simulink model "CIC"  (R2018a)
settings: Solver=ode45  StartTime=0.0  StopTime=Tsim  RelTol=1e-3  EnableMultiTasking=on
values from neighbouring files (symbols this model uses):
  Fin = 15    [Test_CIC.m]
  fo = 10    [Test_CIC.m]
  fsL = 50    [Test_CIC.m]
  M = 1    [Test_CIC.m]
  R = 2000    [Test_CIC.m]
  sel_b = [0 0]    [Test_CIC.m]
  Wg = 22    [Test_CIC.m]
libraries: dspsigops x3, dspsrcs4 x2
settings Model: Creator=jvalls  LastModifiedBy=gsandar
settings DataIOCC: LimitDataPoints=on  SaveFormat=Array  SignalLoggingSaveFormat=ModelDataLogs
settings OptimizationCC: ExpressionDepthLimit=2147483647  LifeSpan=inf
settings DebuggingCC: UnderspecifiedInitializationDetection=Classic  MergeDetectMultiDrivingBlocksExec=none  SolverPrmCheckMsg=warning  ParameterPrecisionLossMsg=none  FcnCallInpInsideContextMsg=warning  StateNameClashWarn=warning  SFUnexpectedBacktrackingDiag=warning  SFNoUnconditionalDefaultTransitionDiag=warning
settings HardwareCC: ProdBitPerPointer=32  ProdBitPerSizeT=32  ProdBitPerPtrDiffT=32  ProdLargestAtomicFloat=None  ProdIntDivRoundTo=Undefined  ProdEndianess=Unspecified  ProdWordSize=32  ProdHWDeviceType=32-bit Generic
settings ModelReferenceCC: PropagateSignalLabelsOutOfModel=off
settings CodeAppCC: StateflowObjectComments=on
settings GRTTargetCC: TargetLangStandard=C89/C90 (ANSI)  CombineOutputUpdateFcns=off  GRTInterface=on
settings ConfigComp: CovMetricSettings=dw  CovSaveCumulativeToWorkspaceVar=on  CovSaveSingleToWorkspaceVar=on  CovExternalEMLEnable=off  CovSFcnEnable=off

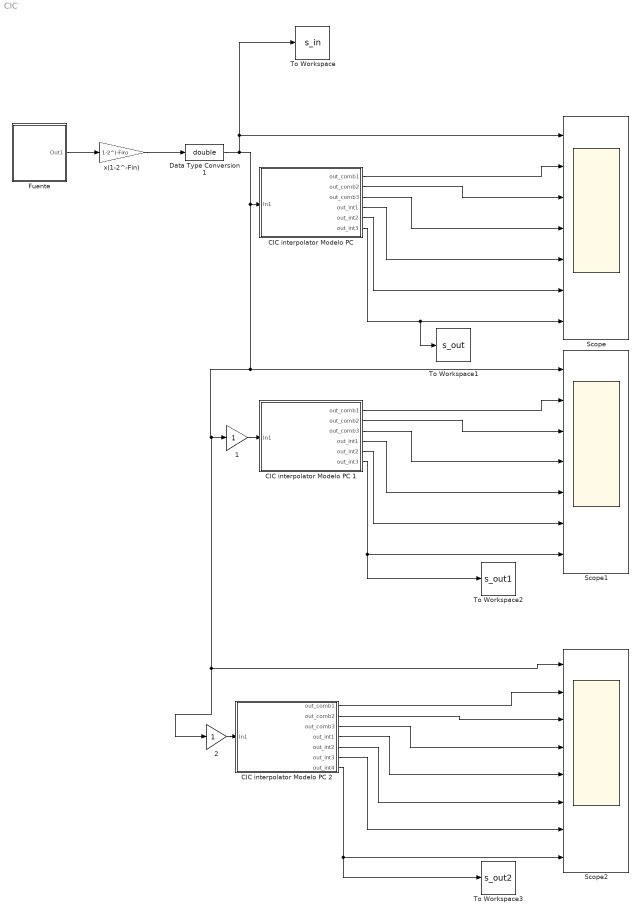
== system CIC ==
  1 : Gain  OutDataTypeStr=fixdt(1,Win,Fin)
  2 : Gain  OutDataTypeStr=fixdt(1,Win,Fin)
  "CIC interpolator Modelo PC " : Subsystem
  CIC interpolator Modelo PC 1 : Subsystem
  CIC interpolator Modelo PC 2 : Subsystem
  Data Type Conversion1 : DataTypeConversion  OutDataTypeStr=double
  Fuente : Subsystem
  Scope : Scope  NumInputPorts=7
  Scope1 : Scope  NumInputPorts=7
  Scope2 : Scope  NumInputPorts=8
  To Workspace : ToWorkspace  VariableName=s_in  SampleTime=-1
      settings: Save2DSignal=2-D array (concatenate along first dimension)
  To Workspace1 : ToWorkspace  VariableName=s_out  SampleTime=-1
      settings: Save2DSignal=2-D array (concatenate along first dimension)
  To Workspace2 : ToWorkspace  VariableName=s_out1  SampleTime=-1
      settings: Save2DSignal=2-D array (concatenate along first dimension)
  To Workspace3 : ToWorkspace  VariableName=s_out2  SampleTime=-1
      settings: Save2DSignal=2-D array (concatenate along first dimension)
  x(1-2^-Fin) : Gain  Gain=1-2^(-Fin)  OutDataTypeStr=fixdt(1,Win,Fin)
  wires:
  Data Type Conversion1/1 -> To Workspace/1, Scope/1, Scope2/1, 2/1, 1/1, Scope1/1, "CIC interpolator Modelo PC "/1(In1)
  Fuente/1(Out1) -> x(1-2^-Fin)/1
  x(1-2^-Fin)/1 -> Data Type Conversion1/1
  "CIC interpolator Modelo PC "/1(out_comb1) -> Scope/2
  "CIC interpolator Modelo PC "/2(out_comb2) -> Scope/3
  "CIC interpolator Modelo PC "/3(out_comb3) -> Scope/4
  "CIC interpolator Modelo PC "/4(out_int1) -> Scope/5
  "CIC interpolator Modelo PC "/5(out_int2) -> Scope/6
  "CIC interpolator Modelo PC "/6(out_int3) -> Scope/7, To Workspace1/1
  CIC interpolator Modelo PC 1/4(out_int1) -> Scope1/5
  CIC interpolator Modelo PC 1/2(out_comb2) -> Scope1/3
  CIC interpolator Modelo PC 1/6(out_int3) -> To Workspace2/1, Scope1/7
  CIC interpolator Modelo PC 1/3(out_comb3) -> Scope1/4
  CIC interpolator Modelo PC 1/1(out_comb1) -> Scope1/2
  CIC interpolator Modelo PC 1/5(out_int2) -> Scope1/6
  1/1 -> CIC interpolator Modelo PC 1/1(In1)
  2/1 -> CIC interpolator Modelo PC 2/1(In1)
  CIC interpolator Modelo PC 2/6(out_int3) -> Scope2/7
  CIC interpolator Modelo PC 2/5(out_int2) -> Scope2/6
  CIC interpolator Modelo PC 2/1(out_comb1) -> Scope2/2
  CIC interpolator Modelo PC 2/2(out_comb2) -> Scope2/3
  CIC interpolator Modelo PC 2/4(out_int1) -> Scope2/5
  CIC interpolator Modelo PC 2/3(out_comb3) -> Scope2/4
  CIC interpolator Modelo PC 2/7(out_int4) -> To Workspace3/1, Scope2/8

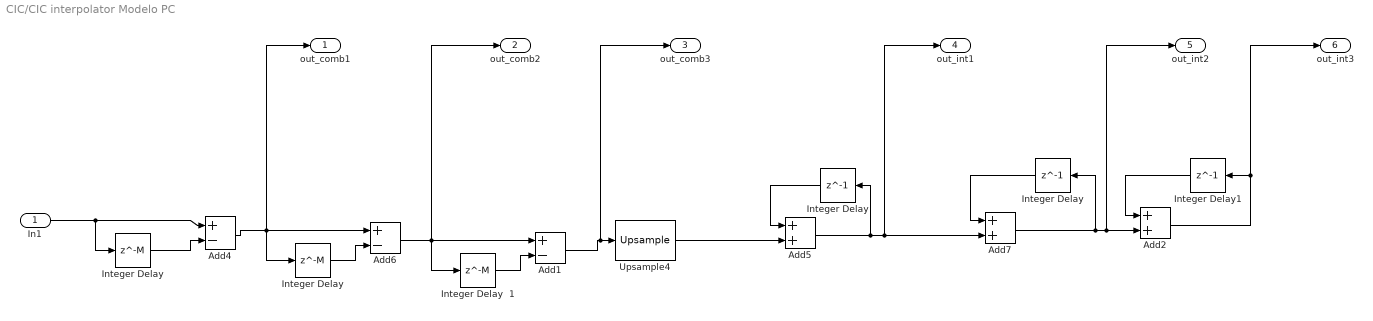
== system CIC/CIC interpolator Modelo PC  ==
  In1 : Inport
  " Integer Delay" : Delay  DelayLength=1
  " Integer Delay1" : Delay  DelayLength=1
  Add1 : Sum  Inputs=+-
  Add2 : Sum
  Add4 : Sum  Inputs=+-
  Add5 : Sum
  Add6 : Sum  Inputs=+-
  Add7 : Sum
  "Integer Delay " : Delay  DelayLength=1
  "Integer Delay " : Delay  DelayLength=M
  "Integer Delay  " : Delay  DelayLength=M
  Integer Delay  1 : Delay  DelayLength=M
  Upsample4 : dspsigops/Upsample  N=R  phase=0  InputProcessing=Columns as channels (frame based)  RateOptions=Allow multirate processing  ic=0  mode=Unused parameter value
  out_comb1 : Outport
  out_comb2 : Outport  Port=2
  out_comb3 : Outport  Port=3
  out_int1 : Outport  Port=4
  out_int2 : Outport  Port=5
  out_int3 : Outport  Port=6
  wires:
  In1/1 -> "Integer Delay "/1, Add4/1
  " Integer Delay"/1 -> Add7/1
  "Integer Delay "/1 -> Add5/1
  "Integer Delay "/1 -> Add4/2
  "Integer Delay  "/1 -> Add6/2
  Integer Delay  1/1 -> Add1/2
  " Integer Delay1"/1 -> Add2/1
  Upsample4/1 -> Add5/2
  Add6/1 -> out_comb2/1, Integer Delay  1/1, Add1/1
  Add4/1 -> out_comb1/1, "Integer Delay  "/1, Add6/1
  Add1/1 -> out_comb3/1, Upsample4/1
  Add5/1 -> "Integer Delay "/1, Add7/2, out_int1/1
  Add7/1 -> out_int2/1, Add2/2, " Integer Delay"/1
  Add2/1 -> out_int3/1, " Integer Delay1"/1

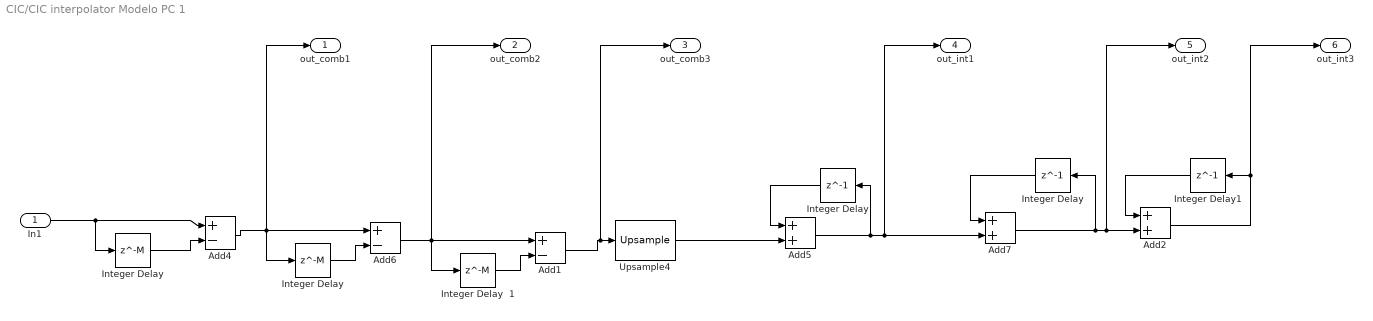
== system CIC/CIC interpolator Modelo PC 1 ==
  In1 : Inport
  " Integer Delay" : Delay  DelayLength=1
  " Integer Delay1" : Delay  DelayLength=1
  Add1 : Sum  Inputs=+-  OutDataTypeStr=fixdt(1,19,15)
  Add2 : Sum  OutDataTypeStr=fixdt(1,38,15)
  Add4 : Sum  Inputs=+-  OutDataTypeStr=fixdt(1,17,15)
  Add5 : Sum  OutDataTypeStr=fixdt(1,38,15)
  Add6 : Sum  Inputs=+-  OutDataTypeStr=fixdt(1,18,15)
  Add7 : Sum  OutDataTypeStr=fixdt(1,38,15)
  "Integer Delay " : Delay  DelayLength=1
  "Integer Delay " : Delay  DelayLength=M
  "Integer Delay  " : Delay  DelayLength=M
  Integer Delay  1 : Delay  DelayLength=M
  Upsample4 : dspsigops/Upsample  N=R  phase=0  InputProcessing=Columns as channels (frame based)  RateOptions=Allow multirate processing  ic=0  mode=Unused parameter value
  out_comb1 : Outport
  out_comb2 : Outport  Port=2
  out_comb3 : Outport  Port=3
  out_int1 : Outport  Port=4
  out_int2 : Outport  Port=5
  out_int3 : Outport  Port=6
  wires:
  In1/1 -> "Integer Delay "/1, Add4/1
  " Integer Delay"/1 -> Add7/1
  "Integer Delay "/1 -> Add5/1
  "Integer Delay "/1 -> Add4/2
  "Integer Delay  "/1 -> Add6/2
  Integer Delay  1/1 -> Add1/2
  " Integer Delay1"/1 -> Add2/1
  Upsample4/1 -> Add5/2
  Add6/1 -> out_comb2/1, Integer Delay  1/1, Add1/1
  Add4/1 -> out_comb1/1, "Integer Delay  "/1, Add6/1
  Add1/1 -> out_comb3/1, Upsample4/1
  Add5/1 -> "Integer Delay "/1, Add7/2, out_int1/1
  Add7/1 -> out_int2/1, Add2/2, " Integer Delay"/1
  Add2/1 -> out_int3/1, " Integer Delay1"/1

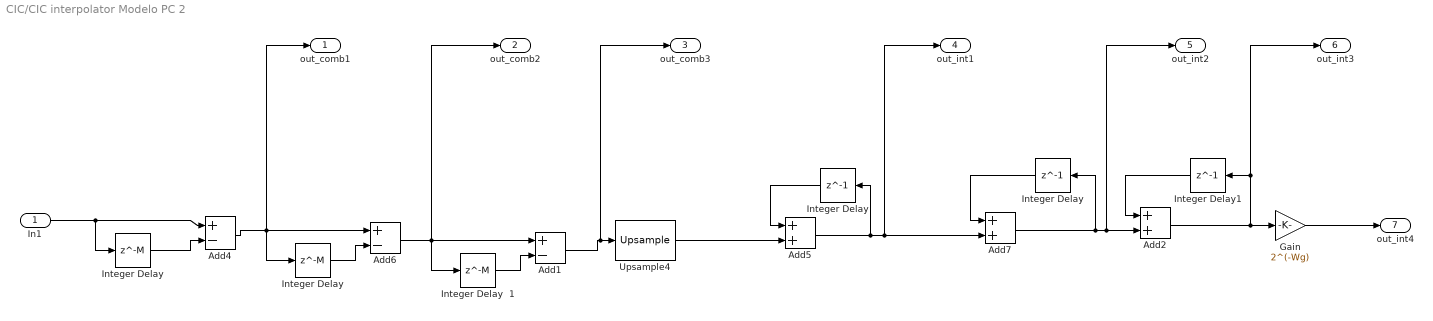
== system CIC/CIC interpolator Modelo PC 2 ==
  In1 : Inport
  " Integer Delay" : Delay  DelayLength=1
  " Integer Delay1" : Delay  DelayLength=1
  Add1 : Sum  Inputs=+-  OutDataTypeStr=fixdt(1,19,15)
  Add2 : Sum  OutDataTypeStr=fixdt(1,38,15)
  Add4 : Sum  Inputs=+-  OutDataTypeStr=fixdt(1,17,15)
  Add5 : Sum  OutDataTypeStr=fixdt(1,38,15)
  Add6 : Sum  Inputs=+-  OutDataTypeStr=fixdt(1,18,15)
  Add7 : Sum  OutDataTypeStr=fixdt(1,38,15)
  Gain : Gain  Gain=2^(-Wg)  OutDataTypeStr=fixdt(1,16,15)
  "Integer Delay " : Delay  DelayLength=1
  "Integer Delay " : Delay  DelayLength=M
  "Integer Delay  " : Delay  DelayLength=M
  Integer Delay  1 : Delay  DelayLength=M
  Upsample4 : dspsigops/Upsample  N=R  phase=0  InputProcessing=Columns as channels (frame based)  RateOptions=Allow multirate processing  ic=0  mode=Unused parameter value
  out_comb1 : Outport
  out_comb2 : Outport  Port=2
  out_comb3 : Outport  Port=3
  out_int1 : Outport  Port=4
  out_int2 : Outport  Port=5
  out_int3 : Outport  Port=6
  out_int4 : Outport  Port=7
  wires:
  In1/1 -> "Integer Delay "/1, Add4/1
  " Integer Delay"/1 -> Add7/1
  "Integer Delay "/1 -> Add5/1
  "Integer Delay "/1 -> Add4/2
  "Integer Delay  "/1 -> Add6/2
  Integer Delay  1/1 -> Add1/2
  " Integer Delay1"/1 -> Add2/1
  Upsample4/1 -> Add5/2
  Add6/1 -> out_comb2/1, Integer Delay  1/1, Add1/1
  Add4/1 -> out_comb1/1, "Integer Delay  "/1, Add6/1
  Add1/1 -> out_comb3/1, Upsample4/1
  Add5/1 -> "Integer Delay "/1, Add7/2, out_int1/1
  Add7/1 -> out_int2/1, Add2/2, " Integer Delay"/1
  Add2/1 -> Gain/1, out_int3/1, " Integer Delay1"/1
  Gain/1 -> out_int4/1

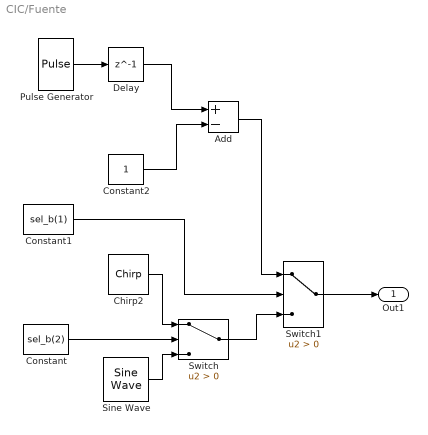
== system CIC/Fuente ==
  Add : Sum  Inputs=+-
  Chirp2 : dspsrcs4/Chirp  sweep=Linear  mode=Unidirectional  f0=5  f1=15*1000  t1=0.001  Tsweep=0.001  phase=0  Ts=1/(fsL*1000)  spf=1  datatype=Double  OutputFrames=on
  Constant : Constant  Value=sel_b(2)
  Constant1 : Constant  Value=sel_b(1)
  Constant2 : Constant
  Delay : Delay  DelayLength=1  InitialCondition=0  SampleTime=1/(fsL*1000)
  Pulse Generator : DiscretePulseGenerator  PulseType=Time based  Amplitude=2  Period=1/(fo*1000)  PulseWidth=50  SampleTime=1/(fsL*1000)
  Sine Wave : dspsrcs4/Sine Wave  Amplitude=1  Frequency=fo*1000  Phase=0  SampleMode=Discrete  OutComplex=Real  CompMethod=Trigonometric fcn  TableSize=Speed  SampleTime=1/(fsL*1000)  SamplesPerFrame=1  ResetState=Restart at time zero  OutputFrames=on  dataType=double  wordLen=16  udDataType=sfix(16)  fracBitsMode=User-defined  numFracBits=15  OutDataTypeStr=double  LastOutDataTypeStr=double
  Switch : Switch  Criteria=u2 > Threshold
  Switch1 : Switch  Criteria=u2 > Threshold
  Out1 : Outport
  wires:
  Constant/1 -> Switch/2
  Switch1/1 -> Out1/1
  Constant1/1 -> Switch1/2
  Sine Wave/1 -> Switch/3
  Chirp2/1 -> Switch/1
  Switch/1 -> Switch1/3
  Add/1 -> Switch1/1
  Constant2/1 -> Add/2
  Delay/1 -> Add/1
  Pulse Generator/1 -> Delay/1
